simulink model "calcul_alpha_beta_gamma"  (R2024b)
settings: Solver=FixedStepAuto  StartTime=0.0  StopTime=10.0  FixedStep=Ts  RelTol=1e-3
settings Model: Creator=marti  LastModifiedBy=Filip

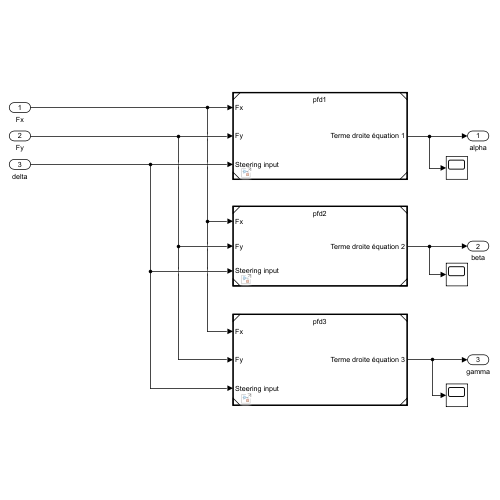
[thumbnail: Simulink's stored preview of the top-level diagram]
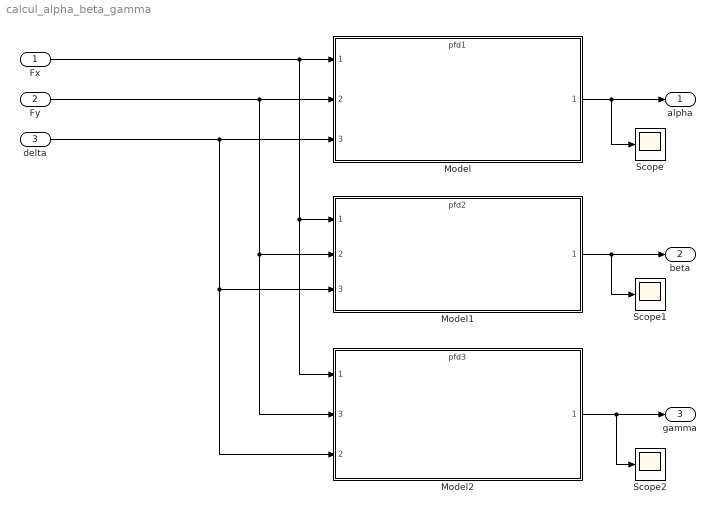
== system calcul_alpha_beta_gamma ==
  Fx : Inport
  Fy : Inport  Port=2
  delta : Inport  Port=3
  Model : ModelReference  ModelNameDialog=pfd1.slx  SimulationMode=Normal  ModelReferenceVersion=1.11
  Model1 : ModelReference  ModelNameDialog=pfd2.slx  SimulationMode=Normal  ModelReferenceVersion=1.5
  Model2 : ModelReference  ModelNameDialog=pfd3.slx  SimulationMode=Normal  ModelReferenceVersion=1.4
      settings: PortSchema="{\"entries\":[{\"content\":{\"sides\":[{\"content\":{\"connectorIds\":[\"In1\",\"In3\",\"In2\"]},\"type\":\"ConnectorPlacement.EquallySpacedRectSide\",\"uuid\":\"32c61a1f-6c57-499a-b866-aceaf52d28d2\"},{\"content\":{\"connectorIds\":[\"Out1\"],\"side\":\"RIGHT\"},\"type\":\"ConnectorPlacement.EquallySpacedRectSide\",\"uuid\":\"cffac577-4d60-419d-9ad2-4916db655c57\"},{\"content\":{\"side\":\"TOP\"},\"type\":\"ConnectorPlacement.EquallySpacedRectSide\",\"uuid\":\"34bdae6d-bec4-41a0-a8ed-c228eaa34691\"}]},\"type\":\"ConnectorPlacement.EquallySpacedConnector\",\"uuid\":\"84af7d52-f463-465c-ba60-2639f593163f\"}],\"packageUris\":[\"http://schema.mathworks.com/mf0/Connector/R2020b\"],\"version\":\"1.0\"}"
  Scope : Scope
  Scope1 : Scope
  Scope2 : Scope
  alpha : Outport
  beta : Outport  Port=2
  gamma : Outport  Port=3
  wires:
  Fx/1 -> Model2/1, Model1/1, Model/1
  Fy/1 -> Model2/3, Model1/2, Model/2
  delta/1 -> Model2/2, Model1/3, Model/3
  Model/1 -> alpha/1, Scope/1
  Model1/1 -> beta/1, Scope1/1
  Model2/1 -> Scope2/1, gamma/1
